simulink model "TCLab_Implementation"  (R2025b)
settings: Solver=FixedStepDiscrete  StartTime=0.0  StopTime=t_final  FixedStep=Ts  RelTol=1e-3  EnableMultiTasking=on
InitFcn:
  | init_TCLab_SIMC
values from neighbouring files (symbols this model uses):
  T_ref = 60    [A8_init_TCLab_SIMC.m]    (also in ELWORKSPACE.mat; SIMC_controller_TCLab.m = str2double(strrep(entrada, ',', '.')); init_TCLab_SIMC.m)
libraries: arduinolib x2, dspstat3 x1
settings Model: SimulationMode=external  SILPILSystemUnderTest=refmodels  ExtModeTrigDuration=2  Creator=jguerrero  LastModifiedBy=matia
settings SolverCC: AutoInsertRateTranBlk=on
settings DataIOCC: ReturnWorkspaceOutputs=off
settings OptimizationCC: EnhancedBackFolding=on  PassReuseOutputArgsAs=Individual arguments  ZeroExternalMemoryAtStartup=off  ZeroInternalMemoryAtStartup=off  MaxStackSize=64  OptimizeBlockOrder=speed  DifferentSizesBufferReuse=on  OptimizationCustomize=off  EfficientTunableParamExpr=on
settings DebuggingCC: UnderspecifiedInitializationDetection=Classic  MergeDetectMultiDrivingBlocksExec=none  ParameterTunabilityLossMsg=error
settings HardwareCC: ProdBitPerInt=16.0  ProdBitPerPointer=16.0  ProdBitPerSizeT=16.0  ProdBitPerPtrDiffT=16.0  ProdLargestAtomicFloat=None  ProdWordSize=8.0  ProdHWDeviceType=Atmel->AVR
settings ModelReferenceCC: PropagateVarSize=During execution  PropagateSignalLabelsOutOfModel=off
settings SFSimCC: MATLABDynamicMemAlloc=off
settings RTWCC: SystemTargetFile=ert.tlc  HardwareBoard=Arduino Leonardo  TemplateMakefile=ert_default_tmf  Toolchain=Arduino AVR  BuildConfiguration=Faster Runs  PortableWordSizes=on  Description=Embedded Coder
settings CodeAppCC: ForceParamTrailComments=on  IgnoreCustomStorageClasses=off  OperatorAnnotations=on  SimulinkDataObjDesc=on  SFDataObjDesc=on  InsertBlockDesc=on
settings ERTTargetCC: ExtModeTransport=3.0  ExtModeStaticAlloc=on  ExtModeAutomaticAllocSize=off  ExtModeStaticAllocSize=250.0  ExtModeMexFile=ext_xcp  ExtModeIntrfLevel=Level2 - Open  InlinedParameterPlacement=Hierarchical  SupportContinuousTime=on  SupportVariableSizeSignals=on

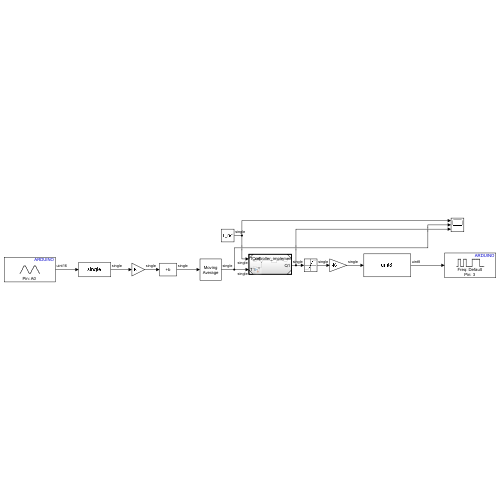
[thumbnail: Simulink's stored preview of the top-level diagram]
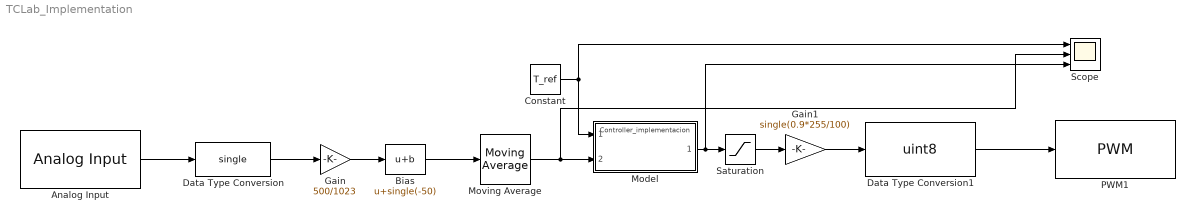
== system TCLab_Implementation ==
  Analog Input : arduinolib/Analog Input  pinNumber=0  ReadResultsOnly=off  ConversionTriggerSource=Software  ExternalTriggerType=uint32( 0 )  OutputDataType=uint16  EnableConversionCompleteNotify=off  EnableOuputStatus=off  SampleTime=-1  blockPlatform=arduino
      settings: LibrarySourceBlock=gizmoLibrary/Arduino Utilities/Analog Input
  Bias : Bias  Bias=single(-50)  SaturateOnIntegerOverflow=off
  Constant : Constant  Value=T_ref  OutDataTypeStr=single
  Data Type Conversion : DataTypeConversion  OutDataTypeStr=single  SaturateOnIntegerOverflow=off  RndMeth=Floor
  Data Type Conversion1 : DataTypeConversion  OutDataTypeStr=uint8  SaturateOnIntegerOverflow=off  RndMeth=Floor
  Gain : Gain  Gain=500/1023
  Gain1 : Gain  Gain=single(0.9*255/100)
  Model : ModelReference  ModelNameDialog=Controller_implementacion  SimulationMode=Normal  ModelReferenceVersion=1.30
  Moving Average : dspstat3/Moving Average  Method=Exponential weighting  ForgettingFactorPort=off  SpecifyWindowLength=on  WindowLength=4  OverlapLength=3  AllowArbitraryInputLength=off  ForgettingFactor=0.5  SimulateUsing=Code generation
  PWM1 : arduinolib/PWM  pinNumber=3  frequencyType=Default  desiredFrequency=50  achievableFrequency=50
      settings: LibrarySourceBlock=gizmoLibrary/Arduino Utilities/PWM
  Saturation : Saturate  UpperLimit=90  LowerLimit=0
  Scope : Scope  NumInputPorts=3
      settings: SampleTime=1  TimeSpan=600  ActiveDisplayYMinimum=2.1083656983653754  ActiveDisplayYMaximum=111.63997107432887
  wires:
  Analog Input/1 -> Data Type Conversion/1
  Data Type Conversion/1 -> Gain/1
  Gain/1 -> Bias/1
  Bias/1 -> Moving Average/1
  Moving Average/1 -> Scope/2, Model/2
  Constant/1 -> Model/1, Scope/1
  Model/1 -> Scope/3, Saturation/1
  Saturation/1 -> Gain1/1
  Gain1/1 -> Data Type Conversion1/1
  Data Type Conversion1/1 -> PWM1/1
